simulink model "FuzzySilmulink1_restored_from_autosave"  (R2022b)
settings: Solver=VariableStepAuto  StartTime=0.0  StopTime=10.0  RelTol=1e-3
libraries: fuzblock x2
settings Model: Creator=user  LastModifiedBy=mluser
settings DebuggingCC: UnconnectedInputMsg=warning  UnconnectedOutputMsg=warning  UnconnectedLineMsg=warning
settings ModelReferenceCC: EnableRefExpFcnMdlSchedulingChecks=on
settings RTWCC: DLArmComputeVersion=19.05

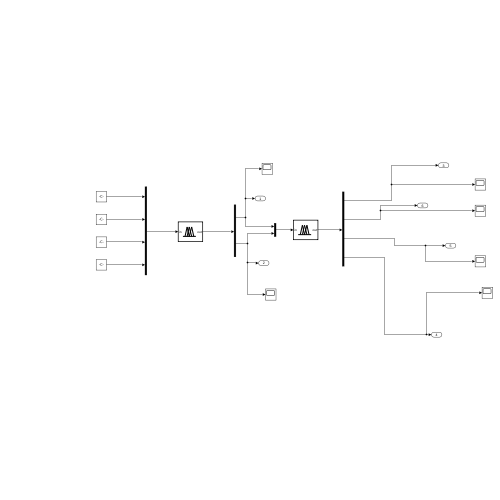
[thumbnail: Simulink's stored preview of the top-level diagram]
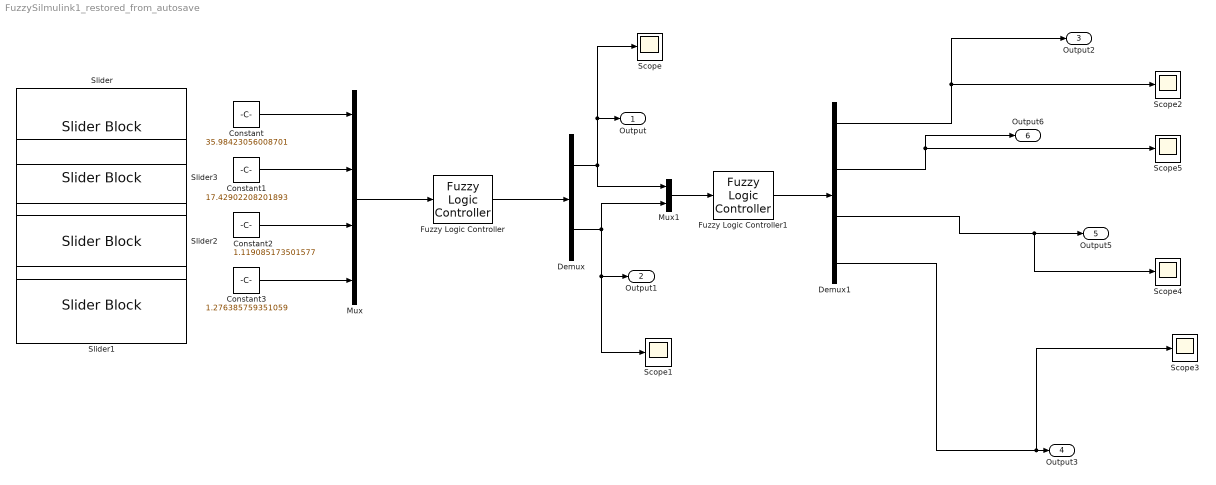
== system FuzzySilmulink1_restored_from_autosave ==
  Constant : Constant  Value=35.98423056008701
  Constant1 : Constant  Value=17.42902208201893
  Constant2 : Constant  Value=1.119085173501577
  Constant3 : Constant  Value=1.276385759351059
  Demux : Demux  Outputs=2
  Demux1 : Demux
  Fuzzy Logic Controller : fuzblock/Fuzzy Logic  Controller  FIS='fuzzy_drone_obstacle.fis'  OutputSampleNumber=101  DataType=double  FuzzifiedInputs=off  RuleFiringStrengths=off  RuleOutputs=off  AggregatedOutputs=off  SimulateUsing=Interpreted execution  OutOfRangeInputValueMessage=warning  NoRuleFiredMessage=warning  EmptyOutputFuzzySetMessage=warning
  Fuzzy Logic Controller1 : fuzblock/Fuzzy Logic  Controller  FIS='MotorFuzzy.fis'  OutputSampleNumber=101  DataType=double  FuzzifiedInputs=off  RuleFiringStrengths=off  RuleOutputs=off  AggregatedOutputs=off  SimulateUsing=Interpreted execution  OutOfRangeInputValueMessage=warning  NoRuleFiredMessage=warning  EmptyOutputFuzzySetMessage=warning
  Mux : Mux
  Mux1 : Mux  Inputs=2
  Scope{,1..5} (6 alike) : Scope
  Slider : SliderBlock  ScaleMax=50
  Slider1 : SliderBlock  ScaleMax=1.8
  Slider2 : SliderBlock  ScaleMax=3.5
  Slider3 : SliderBlock  ScaleMax=50
  Output : Outport
  Output1 : Outport  Port=2
  Output2 : Outport  Port=3
  Output3 : Outport  Port=4
  Output5 : Outport  Port=5
  Output6 : Outport  Port=6
  wires:
  Constant/1 -> Mux/1
  Constant1/1 -> Mux/2
  Constant2/1 -> Mux/3
  Constant3/1 -> Mux/4
  Mux/1 -> Fuzzy Logic Controller/1
  Fuzzy Logic Controller/1 -> Demux/1
  Demux/1 -> Mux1/1, Scope/1, Output/1
  Demux/2 -> Mux1/2, Scope1/1, Output1/1
  Mux1/1 -> Fuzzy Logic Controller1/1
  Fuzzy Logic Controller1/1 -> Demux1/1
  Demux1/1 -> Output2/1, Scope2/1
  Demux1/2 -> Scope5/1, Output6/1
  Demux1/3 -> Scope4/1, Output5/1
  Demux1/4 -> Scope3/1, Output3/1
